simulink model "Transformada_Clarke_Tensao"  (R2014a)
settings: Solver=ode45  StartTime=0.0  StopTime=0.033  MaxStep=1e-4  RelTol=1e-3
settings Model: Creator=Joao  LastModifiedBy=Joao

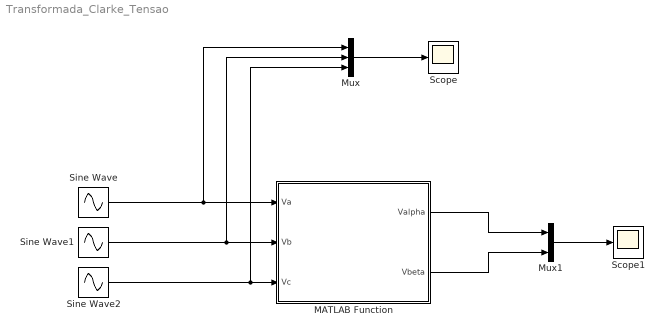
== system Transformada_Clarke_Tensao ==
  MATLAB Function : MATLAB Function  TreatAsAtomicUnit=on
  Mux : Mux  Inputs=3
  Mux1 : Mux  Inputs=2
  Scope : Scope
  Scope1 : Scope
  Sine Wave : Sin  Amplitude=110*sqrt(2)  Frequency=2*pi*60  SampleTime=0
  Sine Wave1 : Sin  Amplitude=110*sqrt(2)  Frequency=2*pi*60  Phase=2*pi/3  SampleTime=0
  Sine Wave2 : Sin  Amplitude=110*sqrt(2)  Frequency=2*pi*60  Phase=-2*pi/3  SampleTime=0
  wires:
  Sine Wave/1 -> Mux/1, MATLAB Function/1(Va)
  Sine Wave1/1 -> Mux/2, MATLAB Function/2(Vb)
  Sine Wave2/1 -> Mux/3, MATLAB Function/3(Vc)
  MATLAB Function/1(Valpha) -> Mux1/1
  MATLAB Function/2(Vbeta) -> Mux1/2
  Mux/1 -> Scope/1
  Mux1/1 -> Scope1/1

== matlab function Transformada_Clarke_Tensao/MATLAB Function ==
  data: Va input; Valpha output; Vb input; Vc input; Vbeta output
function [Valpha,Vbeta] = Transformada_Clarke_Tensao(Va,Vb,Vc)
%#codegen
V = sqrt(2/3)*[1 -1/2 -1/2; 0 sqrt(3)/2 -sqrt(3)/2]*[Va;Vb;Vc]
Valpha = V(1,:);
Vbeta = V(2,:);
